simulink model "FCS"  (R2019b)
settings: Solver=VariableStepAuto  StartTime=0.0  StopTime=10.0  RelTol=1e-3
values from neighbouring files (symbols this model uses):
  a = [1;1]    [MOTIONCONTROL.m]    (also in Robot_Maker.m = evalin('base', 'a'))
  F_v = K_r*diag([0.01 0.01])*K_r    [MOTIONCONTROL.m]
  g = [atan2d(r32,-r31);atan2d(sqrt(power(r13,2)+power(r23,2)),r33);atan2d(r23,r13)]    [DEMOGUI.m]    (also in MOTIONCONTROL.m = 9.81; invJacob_3axis.m = true; inverse_kinematics_Jac.m = true)
  K_d = 750*diag([1 1])    [MOTIONCONTROL.m]
  K_p = 375*diag([1 1])    [MOTIONCONTROL.m]
  pi_l = pi_m    [MOTIONCONTROL.m]
  q_i = [q1ini q2ini]    [MOTIONCONTROL.m]
  Ts = Tc    (= 0.01)    [MOTIONCONTROL.m]
undefined symbols (not defined in the file or in its folder): iner_l
settings Model: Creator=vivek  LastModifiedBy=vivek

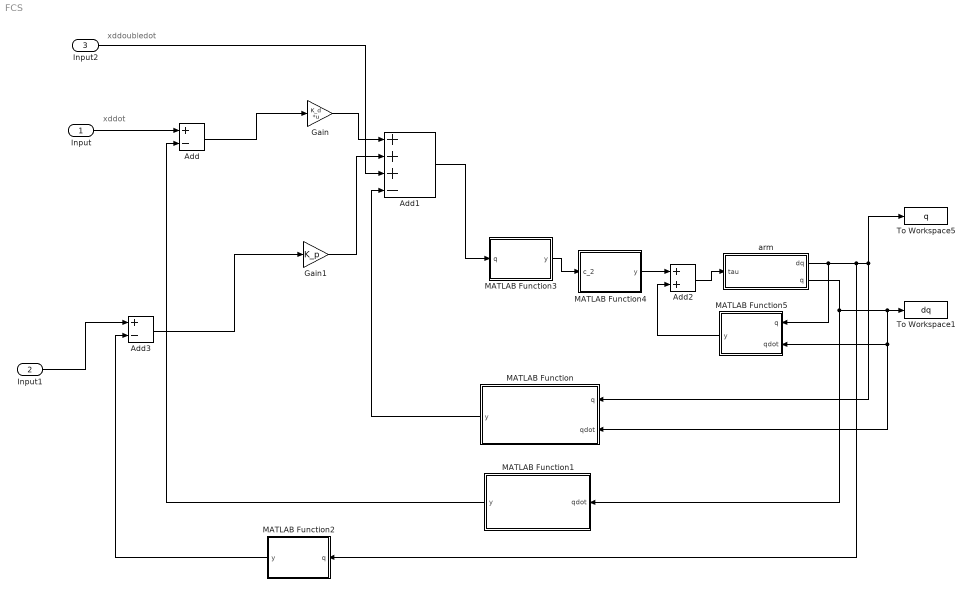
== system FCS ==
  note: xddoubledot
  note: xddot
  Input : Inport
  Input1 : Inport  Port=2
  Input2 : Inport  Port=3
  Add : Sum  Inputs=+-
  Add1 : Sum  Inputs=+++-
  Add2 : Sum
  Add3 : Sum  Inputs=+-
  Gain : Gain  Gain=K_d  Multiplication=Matrix(K*u)
  Gain1 : Gain  Gain=K_p
  MATLAB Function : MATLAB Function  TreatAsAtomicUnit=on
  MATLAB Function1 : MATLAB Function  TreatAsAtomicUnit=on
  MATLAB Function2 : MATLAB Function  TreatAsAtomicUnit=on
  MATLAB Function3 : MATLAB Function  TreatAsAtomicUnit=on
  MATLAB Function4 : MATLAB Function  TreatAsAtomicUnit=on
  MATLAB Function5 : MATLAB Function  TreatAsAtomicUnit=on
  To Workspace1 : ToWorkspace  VariableName=dq  SampleTime=Ts
      settings: MaxDataPoints=4001
  To Workspace5 : ToWorkspace  VariableName=q  SampleTime=Ts
      settings: MaxDataPoints=4001
  arm : Subsystem
      mask Display: disp('inv(B(q))(tau-tau'')')
  wires:
  arm/1(dq) -> MATLAB Function5/1(q), MATLAB Function2/1(q), To Workspace5/1, MATLAB Function/1(q)
  arm/2("q ") -> MATLAB Function1/1(qdot), MATLAB Function5/2(qdot), MATLAB Function/2(qdot), To Workspace1/1
  MATLAB Function/1(y) -> Add1/4
  MATLAB Function1/1(y) -> Add/2
  Add/1 -> Gain/1
  Gain/1 -> Add1/1
  Add1/1 -> MATLAB Function3/1(q)
  MATLAB Function3/1(y) -> MATLAB Function4/1(c_2)
  MATLAB Function4/1(y) -> Add2/1
  Add2/1 -> arm/1(tau)
  Gain1/1 -> Add1/2
  Input/1 -> Add/1
  Input1/1 -> Add3/1
  Add3/1 -> Gain1/1
  MATLAB Function2/1(y) -> Add3/2
  Input2/1 -> Add1/3
  MATLAB Function5/1(y) -> Add2/2

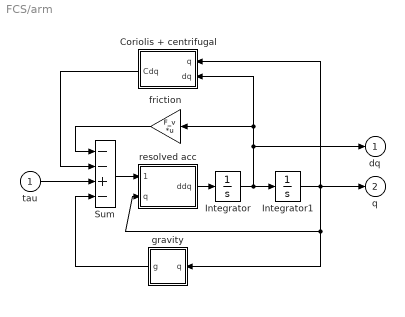
== system FCS/arm ==
  tau : Inport
  Coriolis + centrifugal : Subsystem
      mask Display: disp('C(q,dq)dq')
  Integrator : Integrator  InitialCondition=[0 0]  ZeroCross=off
  Integrator1 : Integrator  InitialCondition=q_i  ZeroCross=off
  Sum : Sum  Inputs=--+-  SaturateOnIntegerOverflow=on  InputSameDT=on  OutDataTypeStr=Inherit: Same as first input
  friction : Gain  Gain=F_v  Multiplication=Matrix(K*u)  SaturateOnIntegerOverflow=on  OutDataTypeStr=Inherit: Same as input  ParamDataTypeStr=Inherit: Same as input
      mask Display: disp('F_v')
  gravity : Subsystem
      mask Display: disp('g(q)')
  resolved acc : Subsystem
      mask Display: disp('inv(B(q))')
  dq : Outport  InitialOutput=0
  "q " : Outport  Port=2  InitialOutput=0
  wires:
  Coriolis + centrifugal/1(Cdq) -> Sum/2
  tau/1 -> Sum/3
  Integrator1/1 -> Coriolis + centrifugal/1(q), resolved acc/2(q), gravity/1(q), "q "/1
  resolved acc/1(ddq) -> Integrator/1
  Integrator/1 -> Integrator1/1, dq/1, Coriolis + centrifugal/2(dq), friction/1
  Sum/1 -> resolved acc/1(tau-tau')
  friction/1 -> Sum/1
  gravity/1(g) -> Sum/4

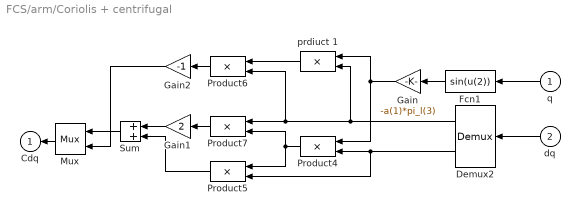
== system FCS/arm/Coriolis + centrifugal ==
  q : Inport
  dq : Inport  Port=2
  Demux2 : Demux  Outputs=2
  Fcn1 : Fcn  Expr=sin(u(2))
  Gain : Gain  Gain=-a(1)*pi_l(3)  SaturateOnIntegerOverflow=on  OutDataTypeStr=Inherit: Same as input  ParamDataTypeStr=Inherit: Same as input
      mask Display: disp('k_3')
  Gain1 : Gain  Gain=2  SaturateOnIntegerOverflow=on  OutDataTypeStr=Inherit: Same as input  ParamDataTypeStr=Inherit: Same as input
  Gain2 : Gain  Gain=-1  SaturateOnIntegerOverflow=on  OutDataTypeStr=Inherit: Same as input  ParamDataTypeStr=Inherit: Same as input
  Mux : Mux  Inputs=2
  Product{4..7} (4 alike) : Product  SaturateOnIntegerOverflow=on  RndMeth=Zero  InputSameDT=on  OutDataTypeStr=Inherit: Same as first input
  Sum : Sum  SaturateOnIntegerOverflow=on  InputSameDT=on  OutDataTypeStr=Inherit: Same as first input
  prdiuct 1 : Product  SaturateOnIntegerOverflow=on  RndMeth=Zero  InputSameDT=on  OutDataTypeStr=Inherit: Same as first input
  Cdq : Outport  InitialOutput=0
  wires:
  dq/1 -> Demux2/1
  Gain2/1 -> Mux/2
  Product6/1 -> Gain2/1
  Mux/1 -> Cdq/1
  Sum/1 -> Mux/1
  Product5/1 -> Sum/2
  Gain1/1 -> Sum/1
  Product7/1 -> Gain1/1
  Demux2/1 -> prdiuct 1/2, Product6/2, Product7/1
  Demux2/2 -> Product4/2, Product5/2
  prdiuct 1/1 -> Product6/1
  Gain/1 -> prdiuct 1/1, Product4/1
  Fcn1/1 -> Gain/1
  q/1 -> Fcn1/1
  Product4/1 -> Product5/1, Product7/2

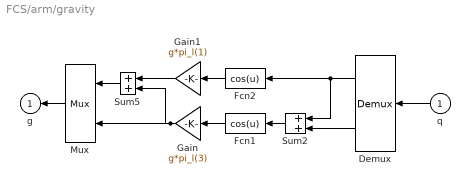
== system FCS/arm/gravity ==
  q : Inport
  Demux : Demux  Outputs=2
  Fcn1 : Fcn  Expr=cos(u)
  Fcn2 : Fcn  Expr=cos(u)
  Gain : Gain  Gain=g*pi_l(3)  SaturateOnIntegerOverflow=on  OutDataTypeStr=Inherit: Same as input  ParamDataTypeStr=Inherit: Same as input
      mask Display: disp('k_2')
  Gain1 : Gain  Gain=g*pi_l(1)  SaturateOnIntegerOverflow=on  OutDataTypeStr=Inherit: Same as input  ParamDataTypeStr=Inherit: Same as input
      mask Display: disp('k_1')
  Mux : Mux  Inputs=2
  Sum2 : Sum  SaturateOnIntegerOverflow=on  InputSameDT=on  OutDataTypeStr=Inherit: Same as first input
  Sum5 : Sum  SaturateOnIntegerOverflow=on  InputSameDT=on  OutDataTypeStr=Inherit: Same as first input
  g : Outport  InitialOutput=0
  wires:
  q/1 -> Demux/1
  Demux/2 -> Sum2/2
  Sum2/1 -> Fcn1/1
  Fcn1/1 -> Gain/1
  Fcn2/1 -> Gain1/1
  Demux/1 -> Fcn2/1, Sum2/1
  Gain1/1 -> Sum5/1
  Sum5/1 -> Mux/1
  Gain/1 -> Sum5/2, Mux/2
  Mux/1 -> g/1

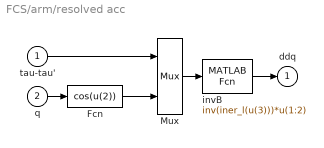
== system FCS/arm/resolved acc ==
  tau-tau' : Inport
  q : Inport  Port=2
  Fcn : Fcn  Expr=cos(u(2))
  Mux : Mux  Inputs=[2,1]
  "invB " : MATLABFcn  MATLABFcn=inv(iner_l(u(3)))*u(1:2)  OutputDimensions=2
      mask Display: disp('inv(B(q))')
  ddq : Outport  InitialOutput=0
  wires:
  Fcn/1 -> Mux/2
  q/1 -> Fcn/1
  "invB "/1 -> ddq/1
  tau-tau'/1 -> Mux/1
  Mux/1 -> "invB "/1

== matlab function FCS/MATLAB Function1 ==
  data: qdot input; y output
function y = alayticaljacobn(qdot)
l1=2;
l2=2;
analytjacobn=[-l1*sin(q(1))-l2*sin(q(1)+q(2)) -l2*sin(q(1)+q(2)); l1*cos(q(1))+l2*(cos(q(1)+cos(2))) l2*cos(q(1)+q(2))];
y = analytjacobn;

== matlab function FCS/MATLAB Function ==
  data: q input; y output; qdot input
function y = analytjacobiandot(q,qdot)
l1=2;
l2=2;
jl11= (-l1*cos(q(1))-l2*cos((q(1)+(q(2)))))*qdot(1)-l2*cos(q(1)+q(2))*qdot(2);
jl12= -l2*cos(q(1)+q(2))*qdot(1)-l2*cos(q(1)+q(2))*qdot(2);
jl21= (-l1*sin(q(1))-l2*sin(q(1)+q(2)))*qdot(1)-l2*sin(q(1)+q(2))*qdot(2);
jl22= -l2*sin(q(1)+q(2))*qdot(1)-l2*sin(q(1)+q(2))*qdot(2);
analyticaljacobdot=[jl11 jl12; jl21 jl22];
y = analyticaljacobdot;

== matlab function FCS/MATLAB Function2 ==
  data: q input; y output
function y = pxpy(q)
l1=2;
l2=2;
px=[l1*cos(q(1))+l2*cos(q(1)+q(2))];
py=[l1*sin(q(1))+l2*sin(q(1)+q(2))];    
y = [px py];

== matlab function FCS/MATLAB Function3 ==
  data: q input; y output
function y = jacobinverse(q)
l1=2;
l2=2;
jl11= -sin(q(1))*l1-l2*sin(q(1)+q(2));
jl12= -l2*sin((q(1)+q(2)));
jl21= l1*cos(q(1))+l2*cos(q(1)+q(2));
jl22= l2*cos(q(1)+q(2));
jacobinverse=inv([jl11 jl12; jl21 jl22]);
y = jacobinverse;

== matlab function FCS/MATLAB Function4 ==
  data: c_2 input; y output
function y = bq(c_2)
global pi_l a k_r2
B=size(2,2);
B(1,1) = a(1)*pi_l(1) + pi_l(2) + (a(2) + 2*a(1)*c_2)*pi_l(3) + pi_l(4);

B(1,2) = (a(2) + a(1)*c_2)*pi_l(3) + pi_l(4) + k_r2*pi_l(5);

B(2,1) = B(1,2);

B(2,2) = a(2)*pi_l(3) + pi_l(4) + k_r2*k_r2*pi_l(5);
y=B;

== matlab function FCS/MATLAB Function5 ==
  data: q input; y output; qdot input
function y = fcn(q,qdot)
Link{1}=Link('d',0,'a',1,'alpha',0,'m',50,'r',[0.5 0 0],'I',[0 0 0;0 10 0; 0 0 0],'G',90,'Jm',0.01);
Link{2}=Link('d',0,'a',1,'alpha',0,'m',50,'r',[0.5 0 0],'I',[0 0 0;0 10 0; 0 0 0],'G',90,'Jm',0.01);
R=SerialLink([Link{1} Link{2}],'name','pro');
C = R.coriolis(q,qdot);
F = R.friction(qdot);
G = R.gravload(q(end,:),[9.8 9.8]);
u=C*qdot+F*qdot+G;
y = u;
